simulink library "nvMemBswLib"  (R2023b)
settings: Solver=VariableStepAuto  StartTime=0.0  StopTime=10.0  RelTol=1e-3
libraries: nvmem_bswapi x2
settings Model: Creator=Professional  LastModifiedBy=Professional
settings SFSimCC: SimUserSources=.\..\..\bswApi\nvmem_bswapi\nvmem_bswapi.cpp  SimAnalyzeCustomCode=on  SimTargetLang=C++
settings SFSimCC: SimCustomHeaderCode=|
  | #include "ecu_types_defines.h"
  | #include "nvmem_bswapi.h"
settings SFSimCC: SimUserIncludeDirs=|
  | .\..\..\bswApi
  | .\..\..\bswApi\nvmem_bswapi
settings RTWCC: RTWUseSimCustomCode=on  CustomSource=.\..\..\bswApi\nvmem_bswapi\nvmem_bswapi.cpp
settings RTWCC: CustomHeaderCode=|
  | #include "ecu_types_defines.h"
  | #include "nvmem_bswapi.h"
settings RTWCC: CustomInclude=|
  | .\..\..\bswApi
  | .\..\..\bswApi\nvmem_bswapi

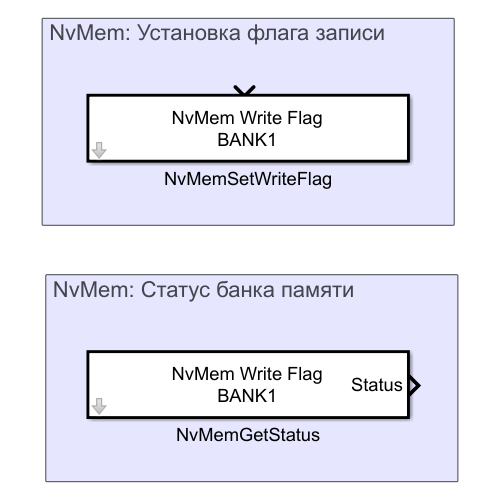
[thumbnail: Simulink's stored preview of the top-level diagram]
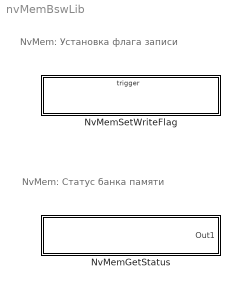
== system nvMemBswLib ==
  note: NvMem: Установка флага записи
  note: NvMem: Статус банка памяти
  NvMemGetStatus : Subsystem  TreatAsAtomicUnit=on  mask(NvMem: GetStatus){bank=BANK1}
      mask prompts: bank "Банк памяти"
      mask help:
      | Проверка статуса ПЗУ
      | Память имеет 4 банка памяти.
      | Status - Enum:Statuses
      mask init:
      | maskObj = Simulink.Mask.get(gcb);
      | bankName = maskObj.getParameter('bank').Value;
      | blockName = "NvMem Write Flag\n" + bankName;
      mask TypeOptions bank: BANK1 | BANK2 | BANK3 | BANK4
      mask DialogControl Container2 Prompt: Параметры:
      mask Display:
      | disp(blockName);
      | port_label('output', 1, 'Status');
  NvMemSetWriteFlag : Subsystem  mask(NvMem: SetWriteFlag){bank=BANK1}
      mask prompts: bank "Банк памяти"
      mask help:
      | Установка флага записи ПЗУ
      | Память имеет 4 банка памяти.
      mask init:
      | maskObj = Simulink.Mask.get(gcb);
      | bankName = maskObj.getParameter('bank').Value;
      | blockName = "NvMem Write Flag\n" + bankName;
      mask TypeOptions bank: BANK1 | BANK2 | BANK3 | BANK4
      mask DialogControl Container2 Prompt: Параметры:
      mask Display: disp(blockName);

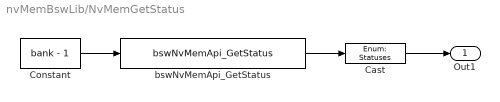
== system nvMemBswLib/NvMemGetStatus ==
  Cast : DataTypeConversion  OutDataTypeStr=Enum: Statuses  RndMeth=Simplest  SaturateOnIntegerOverflow=off
  Constant : Constant  Value=bank - 1  OutDataTypeStr=uint8
  bswNvMemApi_GetStatus : nvmem_bswapi/bswNvMemApi_GetStatus  SampleTime=-1
  Out1 : Outport  OutDataTypeStr=Enum: Statuses
  wires:
  Constant/1 -> bswNvMemApi_GetStatus/1
  bswNvMemApi_GetStatus/1 -> Cast/1
  Cast/1 -> Out1/1

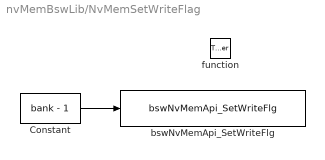
== system nvMemBswLib/NvMemSetWriteFlag ==
  function : TriggerPort  TriggerType=function-call  VariantControl=(inherit)
  Constant : Constant  Value=bank - 1  OutDataTypeStr=uint8
  bswNvMemApi_SetWriteFlg : nvmem_bswapi/bswNvMemApi_SetWriteFlg  SampleTime=-1
  wires:
  Constant/1 -> bswNvMemApi_SetWriteFlg/1
